simulink model "W04_SecondOrder_Sweep"  (R2024b)
settings: Solver=ode45  StartTime=0.0  StopTime=t_end  MaxStep=0.01  RelTol=1e-3
PreLoadFcn:
  | % W04_SecondOrder_Sweep 기본 파라미터 (모델을 열 때 자동 실행)
  | defs = { 'zeta',0.5 ; 'wn',2 ; 't_end',15 };
  | for ii = 1:size(defs,1)
  |     if ~evalin('base', sprintf('exist(''%s'',''var'')', defs{ii,1}))
  |         assignin('base', defs{ii,1}, defs{ii,2});
  |     end
  | end
  | clear defs ii
values from neighbouring files (symbols this model uses):
  wn = 2    [W04_01_first_second_order.m]    (also in W04_03_run_simulink.m)
  zeta = 0    [W04_03_run_simulink.m]
settings Model: Creator=admin  LastModifiedBy=wkyou

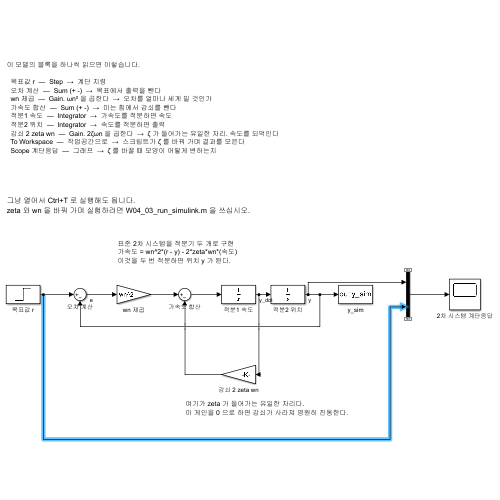
[thumbnail: Simulink's stored preview of the top-level diagram]
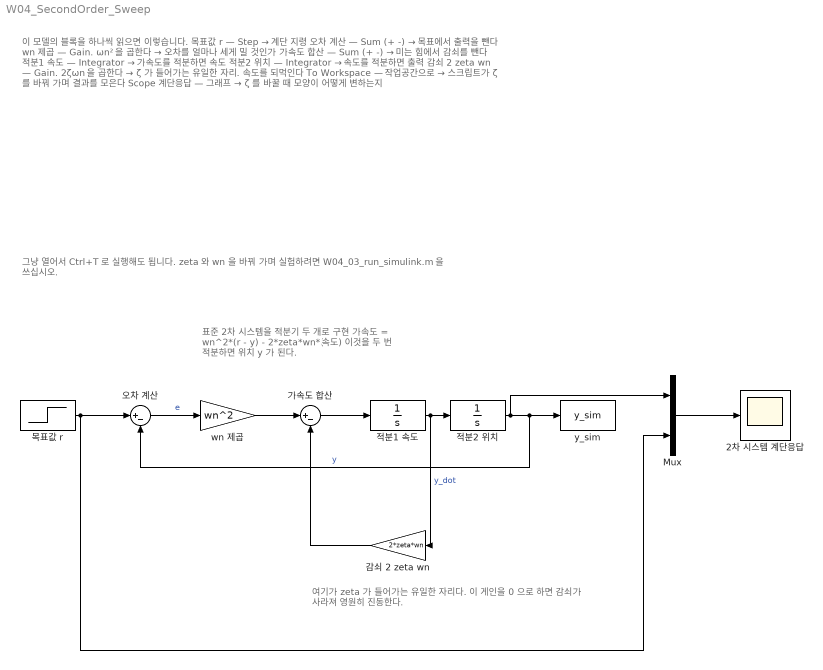
== system W04_SecondOrder_Sweep ==
  note: 표준 2차 시스템을 적분기 두 개로 구현
      | 가속도 = wn^2*(r - y) - 2*zeta*wn*(속도)
      | 이것을 두 번 적분하면 위치 y 가 된다.
  note: 여기가 zeta 가 들어가는 유일한 자리다.
      | 이 게인을 0 으로 하면 감쇠가 사라져 영원히 진동한다.
  note: 그냥 열어서 Ctrl+T 로 실행해도 됩니다.
      | zeta 와 wn 을 바꿔 가며 실험하려면 W04_03_run_simulink.m 을 쓰십시오.
  note: 이 모델의 블록을 하나씩 읽으면 이렇습니다.
      |
      |   목표값 r  —  Step  →  계단 지령
      |   오차 계산  —  Sum (+ -)  →  목표에서 출력을 뺀다
      |   wn 제곱  —  Gain. ωn² 을 곱한다  →  오차를 얼마나 세게 밀 것인가
      |   가속도 합산  —  Sum (+ -)  →  미는 힘에서 감쇠를 뺀다
      |   적분1 속도  —  Integrator  →  가속도를 적분하면 속도
      |   적분2 위치  —  Integrator  →  속도를 적분하면 출력
      |   감쇠 2 zeta wn  —  Gain. 2ζωn 을 곱한다  →  ζ 가 들어가는 유일한 자리. 속도를 되먹인다
      |   To Workspace  —  작업공간으로  →  스크립트가 ζ 를 바꿔 가며 결과를 모은다
      |   Scope 계단응답  —  그래프  →  ζ 를 바꿀 때 모양이 어떻게 변하는지
  2차 시스템 계단응답 : Scope
  Mux : Mux  Inputs=2
  wn 제곱 : Gain  Gain=wn^2
  y_sim : ToWorkspace  VariableName=y_sim  SaveFormat=Timeseries  SampleTime=-1
  가속도 합산 : Sum  Inputs=|+-
  감쇠 2 zeta wn : Gain  Gain=2*zeta*wn
  목표값 r : Step  Time=0  SampleTime=0
  오차 계산 : Sum  Inputs=|+-
  적분1 속도 : Integrator
  적분2 위치 : Integrator
  wires:
  목표값 r/1 -> 오차 계산/1, Mux/2
  오차 계산/1 -> wn 제곱/1  "e"
  wn 제곱/1 -> 가속도 합산/1
  가속도 합산/1 -> 적분1 속도/1
  적분1 속도/1 -> 적분2 위치/1, 감쇠 2 zeta wn/1  "y_dot"
  감쇠 2 zeta wn/1 -> 가속도 합산/2
  적분2 위치/1 -> 오차 계산/2, y_sim/1, Mux/1  "y"
  Mux/1 -> 2차 시스템 계단응답/1
